simulink model "timeDelay_LQR"  (R2022b)
settings: Solver=VariableStepAuto  StartTime=0.0  StopTime=2  RelTol=1e-3
values from neighbouring files (symbols this model uses):
  Aaug = [Ad Bd;zeros(1,3) 0]    [ControllerwithDelay.m]    (also in ControllerwithDelay_LQR.m; ControllerwithDelay_SS.m; DiscreteObserver.m = Ad-Bd)
  Ad = ss_d.A    [ControllerwithDelay.m]    (also in ControllerwithDelay_LQR.m; ControllerwithDelay_PID.m; ControllerwithDelay_SS.m; DiscreteLQControl.m)
  Baug = [0;0;0;1]    [ControllerwithDelay.m]    (also in ControllerwithDelay_LQR.m; ControllerwithDelay_SS.m)
  Bd = ss_d.B    [ControllerwithDelay.m]    (also in ControllerwithDelay_LQR.m; ControllerwithDelay_PID.m; ControllerwithDelay_SS.m; DiscreteLQControl.m)
  Caug = [1 0 0 0]    [ControllerwithDelay.m]    (also in ControllerwithDelay_LQR.m; ControllerwithDelay_SS.m)
  Cd = ss_d.C    [ControllerwithDelay.m]    (also in ControllerwithDelay_LQR.m; ControllerwithDelay_PID.m; ControllerwithDelay_SS.m; DiscreteLQControl.m)
  Klqr_new = place(Aaug,Baug,[-0.4 -0.5069+0.2i -0.5069-0.2i -0.1])    [ControllerwithDelay_LQR.m]
undefined symbols (not defined in the file or in its folder): Klqr_old, Klqr_old2
settings Model: Creator=1  LastModifiedBy=DAVID CHEN
settings ModelReferenceCC: EnableRefExpFcnMdlSchedulingChecks=on

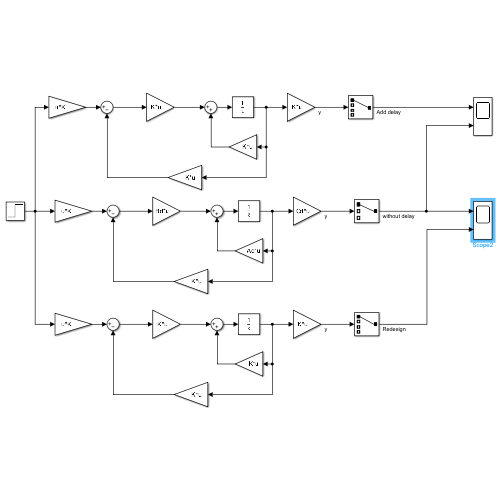
[thumbnail: Simulink's stored preview of the top-level diagram]
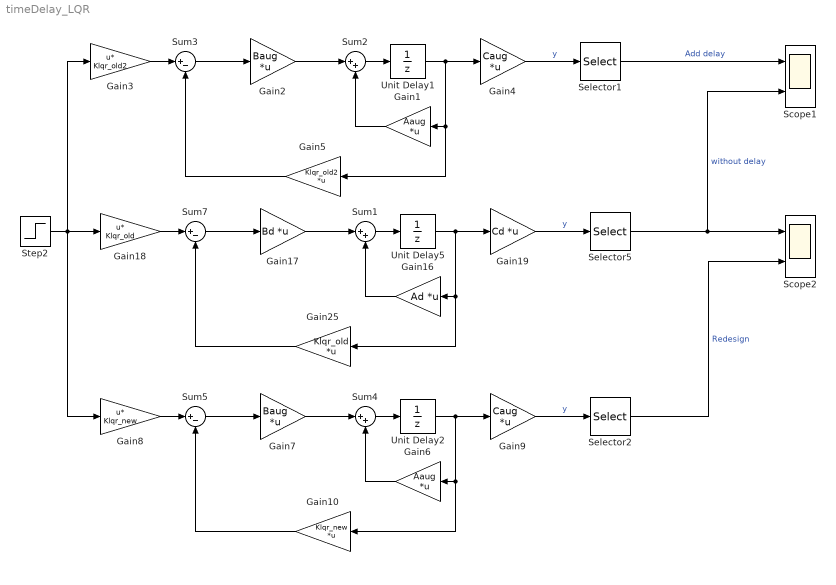
== system timeDelay_LQR ==
  Gain1 : Gain  Gain=Aaug  Multiplication=Matrix(K*u)
  Gain10 : Gain  Gain=Klqr_new  Multiplication=Matrix(K*u)
  Gain16 : Gain  Gain=Ad  Multiplication=Matrix(K*u)
  Gain17 : Gain  Gain=Bd  Multiplication=Matrix(K*u)
  Gain18 : Gain  Gain=Klqr_old  Multiplication=Matrix(u*K)
  Gain19 : Gain  Gain=Cd  Multiplication=Matrix(K*u)
  Gain2 : Gain  Gain=Baug  Multiplication=Matrix(K*u)
  Gain25 : Gain  Gain=Klqr_old  Multiplication=Matrix(K*u)
  Gain3 : Gain  Gain=Klqr_old2  Multiplication=Matrix(u*K)
  Gain4 : Gain  Gain=Caug  Multiplication=Matrix(K*u)
  Gain5 : Gain  Gain=Klqr_old2  Multiplication=Matrix(K*u)
  Gain6 : Gain  Gain=Aaug  Multiplication=Matrix(K*u)
  Gain7 : Gain  Gain=Baug  Multiplication=Matrix(K*u)
  Gain8 : Gain  Gain=Klqr_new  Multiplication=Matrix(u*K)
  Gain9 : Gain  Gain=Caug  Multiplication=Matrix(K*u)
  Scope1 : Scope  NumInputPorts=2
  Scope2 : Scope  NumInputPorts=2
  Selector1 : Selector  InputPortWidth=4  IndexOptions=Index vector (dialog)  Indices=[1]  OutputSizes=1
  Selector2 : Selector  InputPortWidth=4  IndexOptions=Index vector (dialog)  Indices=[1]  OutputSizes=1
  Selector5 : Selector  InputPortWidth=3  IndexOptions=Index vector (dialog)  Indices=[1]  OutputSizes=1
  Step2 : Step  Time=0.1  SampleTime=0
  Sum1 : Sum  Inputs=|++
  Sum2 : Sum  Inputs=|++
  Sum3 : Sum  Inputs=|+-
  Sum4 : Sum  Inputs=|++
  Sum5 : Sum  Inputs=|+-
  Sum7 : Sum  Inputs=|+-
  Unit Delay1 : UnitDelay  SampleTime=-1  HasFrameUpgradeWarning=on
  Unit Delay2 : UnitDelay  SampleTime=-1  HasFrameUpgradeWarning=on
  Unit Delay5 : UnitDelay  SampleTime=-1  HasFrameUpgradeWarning=on
  wires:
  Step2/1 -> Gain8/1, Gain3/1, Gain18/1
  Gain17/1 -> Sum1/1
  Gain19/1 -> Selector5/1  "y"
  Sum1/1 -> Unit Delay5/1
  Gain25/1 -> Sum7/2
  Gain16/1 -> Sum1/2
  Unit Delay5/1 -> Gain16/1, Gain25/1, Gain19/1
  Gain18/1 -> Sum7/1
  Sum7/1 -> Gain17/1
  Selector5/1 -> Scope1/2, Scope2/1  "without delay"
  Sum3/1 -> Gain2/1
  Gain5/1 -> Sum3/2
  Gain1/1 -> Sum2/2
  Gain3/1 -> Sum3/1
  Unit Delay1/1 -> Gain1/1, Gain5/1, Gain4/1
  Gain4/1 -> Selector1/1  "y"
  Gain2/1 -> Sum2/1
  Sum2/1 -> Unit Delay1/1
  Selector1/1 -> Scope1/1  "Add delay"
  Sum4/1 -> Unit Delay2/1
  Unit Delay2/1 -> Gain6/1, Gain10/1, Gain9/1
  Gain7/1 -> Sum4/1
  Gain9/1 -> Selector2/1  "y"
  Gain8/1 -> Sum5/1
  Gain6/1 -> Sum4/2
  Sum5/1 -> Gain7/1
  Gain10/1 -> Sum5/2
  Selector2/1 -> Scope2/2  "Redesign"
